simulink model "simulacion_un_tanque"  (R2015b)
settings: Solver=VariableStepAuto  StartTime=0.0  StopTime=25.0  RelTol=1e-3
settings Model: Creator=nico  LastModifiedBy=nico

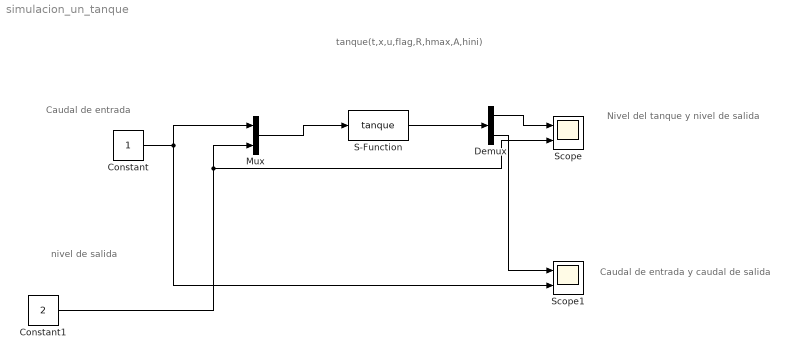
== system simulacion_un_tanque ==
  note: tanque(t,x,u,flag,R,hmax,A,hini)
  note: nivel de salida
  note: Caudal de entrada
  note: Caudal de entrada y caudal de salida
  note: Nivel del tanque y nivel de salida
  Constant : Constant
  Constant1 : Constant  Value=2
  Demux : Demux  Outputs=2
  Mux : Mux  Inputs=2
  S-Function : S-Function  FunctionName=tanque  Parameters=1 8 1 5  SFunctionDeploymentMode=off  EnableBusSupport=off
  Scope : Scope  NumInputPorts=2
  Scope1 : Scope  NumInputPorts=2
  wires:
  Constant/1 -> Mux/1, Scope1/2
  Mux/1 -> S-Function/1
  S-Function/1 -> Demux/1
  Demux/1 -> Scope/1
  Demux/2 -> Scope1/1
  Constant1/1 -> Scope/2, Mux/2
